simulink model "StdAnimation"  (R2020b)
settings: configuration reference "VLS_Standard_Configuration" (kept outside this file)
undefined symbols (not defined in the file): C_AnimationOnLoop, C_AnimationPeriod, C_CieCurveGammaToPwmY, C_CieCurvePwmToGammaY, C_DefaultValue, C_EndValues, C_IndexOfStartStepForEachScenario, C_MaintainAnimationPwm, C_MaintainAnimationTime, C_NumOfStepsForEachScenario, C_StartValues, C_TRamp, C_TStart
libraries: StdAnimationLibrary_R2020b x1
settings Model: DataDictionary=StdAnimation_DD.sldd  Creator=mchawa  LastModifiedBy=oashraf
settings ConfigSetRef: SourceName=VLS_Standard_Configuration

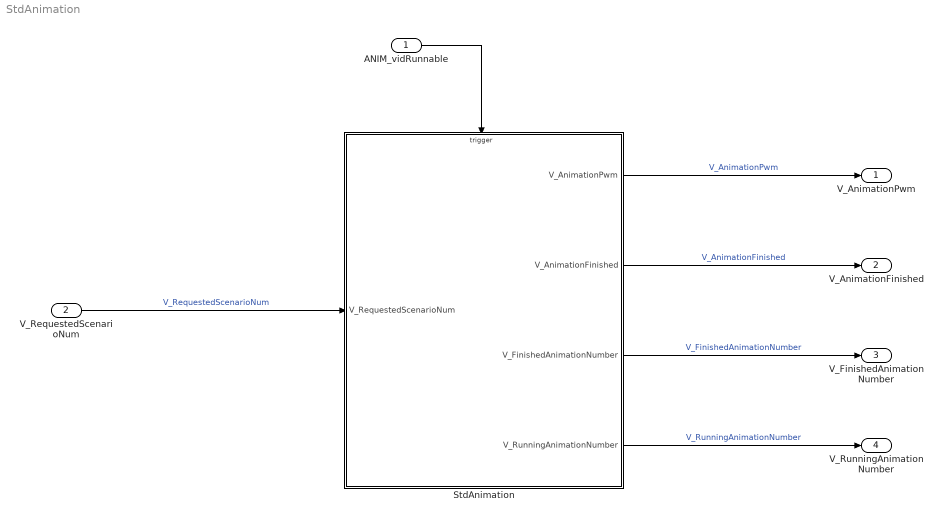
== system StdAnimation ==
  ANIM_vidRunnable : Inport  OutputFunctionCall=on
  V_RequestedScenarioNum : Inport  Port=2
  StdAnimation : Subsystem  TreatAsAtomicUnit=on
  V_AnimationPwm : Outport
  V_AnimationFinished : Outport  Port=2
  V_FinishedAnimationNumber : Outport  Port=3
  V_RunningAnimationNumber : Outport  Port=4
  wires:
  StdAnimation/4(V_RunningAnimationNumber) -> V_RunningAnimationNumber/1  "V_RunningAnimationNumber"
  StdAnimation/3(V_FinishedAnimationNumber) -> V_FinishedAnimationNumber/1  "V_FinishedAnimationNumber"
  StdAnimation/2(V_AnimationFinished) -> V_AnimationFinished/1  "V_AnimationFinished"
  StdAnimation/1(V_AnimationPwm) -> V_AnimationPwm/1  "V_AnimationPwm"
  V_RequestedScenarioNum/1 -> StdAnimation/1(V_RequestedScenarioNum)  "V_RequestedScenarioNum"
  ANIM_vidRunnable/1 -> StdAnimation/Trigger

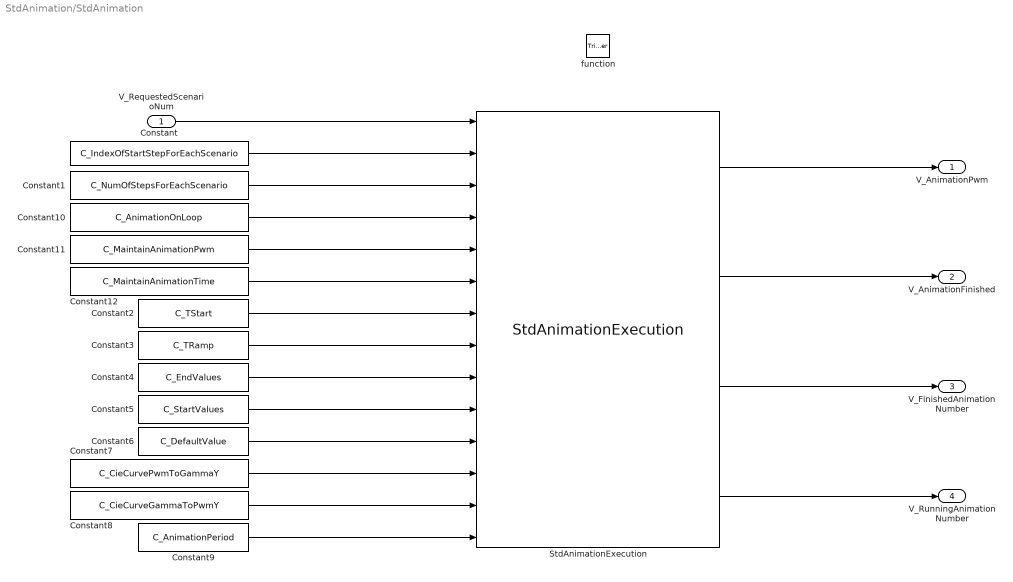
== system StdAnimation/StdAnimation ==
  V_RequestedScenarioNum : Inport
  function : TriggerPort  TriggerType=function-call  VariantControl=Variant
  Constant : Constant  Value=C_IndexOfStartStepForEachScenario  VectorParams1D=off
  Constant1 : Constant  Value=C_NumOfStepsForEachScenario  VectorParams1D=off
  Constant10 : Constant  Value=C_AnimationOnLoop  OutDataTypeStr=uint8
  Constant11 : Constant  Value=C_MaintainAnimationPwm  OutDataTypeStr=uint8
  Constant12 : Constant  Value=C_MaintainAnimationTime
  Constant2 : Constant  Value=C_TStart
  Constant3 : Constant  Value=C_TRamp
  Constant4 : Constant  Value=C_EndValues
  Constant5 : Constant  Value=C_StartValues  VectorParams1D=off
  Constant6 : Constant  Value=C_DefaultValue  OutDataTypeStr=uint8
  Constant7 : Constant  Value=C_CieCurvePwmToGammaY
  Constant8 : Constant  Value=C_CieCurveGammaToPwmY
  Constant9 : Constant  Value=C_AnimationPeriod
  StdAnimationExecution : StdAnimationLibrary_R2020b/StdAnimationExecution  Description=|  SystemSampleTime=-1  VariantActivationTime=update diagram  Latency=0  AutoFrameSizeCalculation=off
      | S___122_135
      | S___122_242
      | S___122_240
  V_AnimationPwm : Outport
  V_AnimationFinished : Outport  Port=2
  V_FinishedAnimationNumber : Outport  Port=3
  V_RunningAnimationNumber : Outport  Port=4
  wires:
  Constant3/1 -> StdAnimationExecution/8
  StdAnimationExecution/2 -> V_AnimationFinished/1
  StdAnimationExecution/4 -> V_RunningAnimationNumber/1
  StdAnimationExecution/1 -> V_AnimationPwm/1
  Constant4/1 -> StdAnimationExecution/9
  Constant2/1 -> StdAnimationExecution/7
  Constant1/1 -> StdAnimationExecution/3
  Constant9/1 -> StdAnimationExecution/14
  Constant5/1 -> StdAnimationExecution/10
  Constant11/1 -> StdAnimationExecution/5
  V_RequestedScenarioNum/1 -> StdAnimationExecution/1
  Constant10/1 -> StdAnimationExecution/4
  Constant12/1 -> StdAnimationExecution/6
  Constant6/1 -> StdAnimationExecution/11
  StdAnimationExecution/3 -> V_FinishedAnimationNumber/1
  Constant/1 -> StdAnimationExecution/2
  Constant8/1 -> StdAnimationExecution/13
  Constant7/1 -> StdAnimationExecution/12
